simulink model "KalmanPrep"  (R2023b)
settings: Solver=FixedStepAuto  StartTime=0.0  StopTime=50  FixedStep=0.001  RelTol=1e-3
values from neighbouring files (symbols this model uses):
  A = [1, 0, Ts, 0 ... (first row only)    [Kal5Prep.m]    (also in KalPrep_mat.m = [1, Ts)
  B = [Ts, 0 ... (first row only)    [Kal5Prep.m]    (also in KalPrep_mat.m = [Ts; 0])
  bias = 0.5    [KalPrep_mat.m]
  C = [1, 0]    [KalPrep_mat.m]
  cov_ic = P0 * (1 + 2*rand)    [Kal5Prep.m]    (also in KalPrep_mat.m = eye(2) * alpha)
  eta1 = 0.002    [Kal5Prep.m]    (also in KalPrep_mat.m = deg2rad(1))
  eta2 = 0    [KalPrep_mat.m]
  eta_max = 0.4    [KalPrep_mat.m]
  G = eye(4) * Ts    [Kal5Prep.m]    (also in KalPrep_mat.m = [Ts 0)
  init_cond = [0; 0; 0.02; 0.01]    [Kal5Prep.m]    (also in KalPrep_mat.m = [pi/2; 5])
  K1 = 0.48    [KalPrep_mat.m]
  K2 = 0.16    [KalPrep_mat.m]
  pb = [0.5; 0.5]    [Kal5Prep.m]
  Q = eye(4)    [Kal5Prep.m]    (also in KalPrep_mat.m = [(sig1^2), 0)
  R = (eta1)^2    (= 4e-06)    [Kal5Prep.m]    (also in KalPrep_mat.m = (eta1)^2)
  sig1 = 0.005    [Kal5Prep.m]    (also in KalPrep_mat.m = 0.1)
  sig2 = 0.001    [Kal5Prep.m]    (also in KalPrep_mat.m = 0.2)
  Ts = 0.001    [Kal5Prep.m]    (also in KalPrep_mat.m)
  v0 = [1; 0]    [Kal5Prep.m]
libraries: dspsrcs4 x3
settings Model: Creator=fabio  LastModifiedBy=fabio

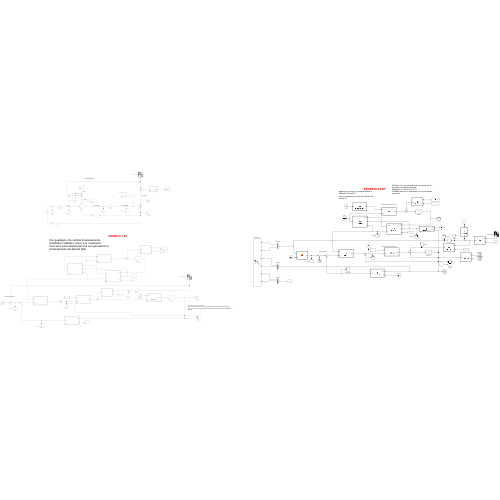
[thumbnail: Simulink's stored preview of the top-level diagram]
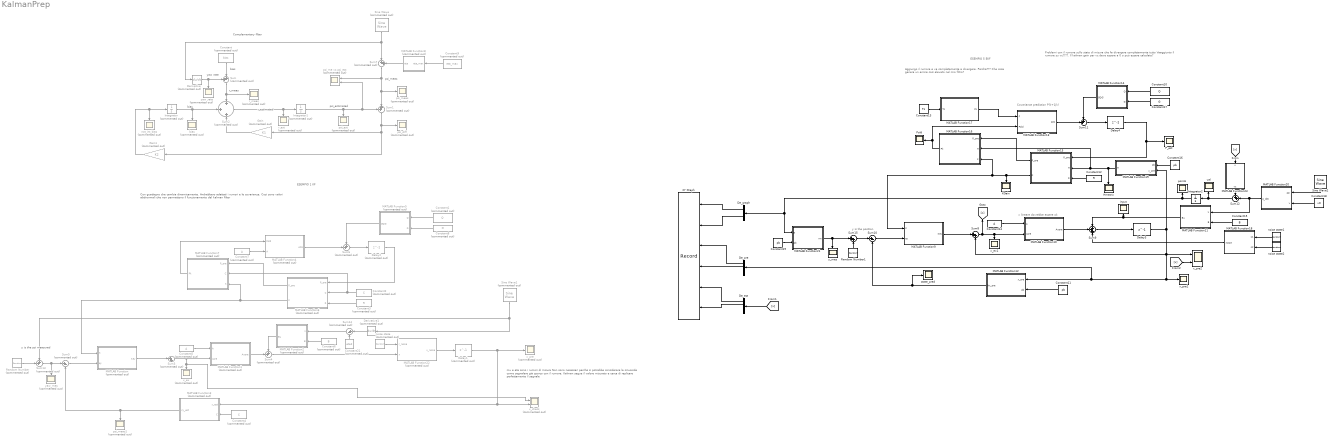
== system KalmanPrep ==
  note: Problemi con il rumore sullo stato di misura che fa divergere completamente tutto
      | Vaaggiunto il rumore su vc????.
      | Il kalman gain per vc deve essere a 0 o può essere calcolato?
  note: Aggiungo il rumore e va completamente a divergere. Perchè???
      | Che cosa genera un errore così elevato nel mio filtro?
  note: Complementary filter
  note: mu e eta sono i rumori di misura
      | Non sono necessari perchè si potrebbe considerare la sinusoide come segnalere già sporco con il rumore. Kalman segue il valore misurato e cerca di replicare perfettamente il segnale
  note: x lineare dovrebbe essere ok
  note: Covariance prediction P(k+1|k)
  note: ESEMPIO 5 EKF
  note: ESEMPIO 1 KF
  note: Con guadagno che cambia dinamicamente.
      | Andrebbero adattati i rumori e le covarianze.
      | Così sono valori abdnormali che non permettono il funzionamento del kalman filter
  note: y is the psi measured
  note: psi_meas
  note: yaw rate
  note: bias
  note: r_meas
  note: bias
  note: r_estimated
  note: psi_estimated
  note: y is the position
  Constant : Constant  Commented=on  Value=bias
  Constant1 : Constant  Commented=on  Value=Q
  Constant10 : Constant  Value=Q  VectorParams1D=off
  Constant11 : Constant  Value=pb  VectorParams1D=off
  Constant12 : Constant  Value=R
  Constant13 : Constant  Value=Ts
  Constant14 : Constant  Value=A  VectorParams1D=off
  Constant15 : Constant  Value=B  VectorParams1D=off
  Constant16 : Constant  Value=pb  VectorParams1D=off
  Constant17 : Constant  Value=G  VectorParams1D=off
  Constant18 : Constant  Value=v0  VectorParams1D=off
  Constant19 : Constant  Value=pb  VectorParams1D=off
  Constant2 : Constant  Commented=on  Value=C  VectorParams1D=off
  Constant21 : Constant  Commented=on  Value=eta2  VectorParams1D=off
  Constant3 : Constant  Commented=on  Value=R
  Constant4 : Constant  Commented=on  Value=C  VectorParams1D=off
  Constant5 : Constant  Commented=on  Value=A
  Constant6 : Constant  Commented=on  Value=B
  Constant7 : Constant  Commented=on  Value=A
  Constant8 : Constant  Commented=on  Value=G
  Constant9 : Constant  Commented=on  Value=eta_max
  De_est : Demux
  De_graph : Demux  Outputs=2
  De_pre : Demux
  Delay1 : Delay  Commented=on  DelayLength=1  InitialCondition=init_cond  UseCircularBuffer=on
  Delay2 : Delay  Commented=on  DelayLength=1  InitialCondition=cov_ic  UseCircularBuffer=on
  Delay3 : Delay  DelayLength=1  InitialCondition=init_cond  UseCircularBuffer=on
  Delay4 : Delay  DelayLength=1  InitialCondition=cov_ic  UseCircularBuffer=on
  Derivative : Derivative  Commented=on
  Derivative1 : Derivative  Commented=on
  Gain : Gain  Commented=on  Gain=K1
  Gain1 : Gain  Commented=on  Gain=K2
  Hmatrix : Scope
  Integrator : Integrator  Commented=on
  Integrator1 : Integrator  Commented=on
  Integrator2 : Integrator
  KGain : Scope
  MATLAB Function : MATLAB Function  Commented=on  TreatAsAtomicUnit=on
  MATLAB Function1 : MATLAB Function  Commented=on  TreatAsAtomicUnit=on
  MATLAB Function10 : MATLAB Function  TreatAsAtomicUnit=on
  MATLAB Function11 : MATLAB Function  TreatAsAtomicUnit=on
  MATLAB Function12 : MATLAB Function  TreatAsAtomicUnit=on
  MATLAB Function13 : MATLAB Function  TreatAsAtomicUnit=on
  MATLAB Function14 : MATLAB Function  TreatAsAtomicUnit=on
  MATLAB Function15 : MATLAB Function  TreatAsAtomicUnit=on
  MATLAB Function16 : MATLAB Function  TreatAsAtomicUnit=on
  MATLAB Function17 : MATLAB Function  TreatAsAtomicUnit=on
  MATLAB Function18 : MATLAB Function  TreatAsAtomicUnit=on
  MATLAB Function19 : MATLAB Function  TreatAsAtomicUnit=on
  MATLAB Function2 : MATLAB Function  Commented=on  TreatAsAtomicUnit=on
  MATLAB Function20 : MATLAB Function  TreatAsAtomicUnit=on
  MATLAB Function21 : MATLAB Function  TreatAsAtomicUnit=on
  MATLAB Function22 : MATLAB Function  Commented=on  TreatAsAtomicUnit=on
  MATLAB Function23 : MATLAB Function  TreatAsAtomicUnit=on
  MATLAB Function3 : MATLAB Function  Commented=on  TreatAsAtomicUnit=on
  MATLAB Function4 : MATLAB Function  Commented=on  TreatAsAtomicUnit=on
  MATLAB Function5 : MATLAB Function  Commented=on  TreatAsAtomicUnit=on
  MATLAB Function6 : MATLAB Function  Commented=on  TreatAsAtomicUnit=on
  MATLAB Function7 : MATLAB Function  Commented=on  TreatAsAtomicUnit=on
  MATLAB Function8 : MATLAB Function  Commented=on  TreatAsAtomicUnit=on
  MATLAB Function9 : MATLAB Function  TreatAsAtomicUnit=on
  P_est : Scope
  Pold : Scope
  Random Number : RandomNumber  Commented=on  Variance=eta1  SampleTime=Ts  VectorParams1D=off
  Random Number1 : RandomNumber  Variance=eta1  SampleTime=Ts
  Sine Wave : dspsrcs4/Sine Wave  Commented=on  Amplitude=1  Frequency=100  Phase=0  SampleMode=Discrete  OutComplex=Real  CompMethod=Trigonometric fcn  TableSize=Speed  SampleTime=1/1000  SamplesPerFrame=1  ResetState=Restart at time zero  OutputFrames=off  dataType=double  wordLen=16  udDataType=sfix(16)  fracBitsMode=Best precision  numFracBits=15  OutDataTypeStr=double  LastOutDataTypeStr=double
  Sine Wave1 : dspsrcs4/Sine Wave  Commented=on  Amplitude=1  Frequency=10  Phase=0  SampleMode=Discrete  OutComplex=Real  CompMethod=Trigonometric fcn  TableSize=Speed  SampleTime=1/1000  SamplesPerFrame=1  ResetState=Restart at time zero  OutputFrames=off  dataType=double  wordLen=16  udDataType=sfix(16)  fracBitsMode=Best precision  numFracBits=15  OutDataTypeStr=double  LastOutDataTypeStr=double
  Sine Wave2 : dspsrcs4/Sine Wave  Amplitude=1  Frequency=0.1  Phase=0  SampleMode=Discrete  OutComplex=Real  CompMethod=Trigonometric fcn  TableSize=Speed  SampleTime=1/1000  SamplesPerFrame=1  ResetState=Restart at time zero  OutputFrames=off  dataType=double  wordLen=16  udDataType=sfix(16)  fracBitsMode=Best precision  numFracBits=15  OutDataTypeStr=double  LastOutDataTypeStr=double
  Sum{,1,4,6,13} (5 alike) : Sum  Commented=on  Inputs=++|
  Sum10 : Sum  Inputs=|+-
  Sum11 : Sum  Inputs=++|
  Sum12 : Sum  Inputs=++|
  Sum14 : Sum  Commented=on  Inputs=|+-
  Sum15 : Sum  Inputs=|++
  Sum2 : Sum  Commented=on  Inputs=+||+||+
  Sum3 : Sum  Commented=on  Inputs=|++
  Sum5 : Sum  Commented=on  Inputs=|+-
  Sum7 : Sum  Commented=on  Inputs=|++
  Sum8 : Sum  Inputs=|++
  Sum9 : Sum  Inputs=+++
  XY Graph : Record  FileSettingsInternal="{\"entries\":[{\"content\":{\"excelSettings\":{\"content\":{},\"type\":\"Streamout.ExcelSettings\"}},\"type\":\"Streamout.FileSettingStorage\",\"uuid\":\"\"}],\"packageUris\":[\"http:\\/\\/schema.mathworks.com\\/mf0\\/streamout_blocks\\/R2020a\"],\"version\":\"1.0\"}"  Layout=[1 1]  SignalsInternal="{\"entries\":[{\"content\":{\"signals\":[{\"content\":{\"blockPath\":[],\"dimensions\":[1],\"domain\":\"\",\"lineColor\":\"#fe330a\",\"plots\":[ 1 ],\"port\":1,\"sid\":[\"\"],\"signalID\":1,\"signalName\":\"De_graph:1\"},\"type\":\"RecordBlkView.Signal\",\"uuid\":\"\"},{\"content\":{\"blockPath\":[],\"dimensions\":[1],\"domain\":\"\",\"lineColor\":\"#d95319\",\"plots\":[ 1 ],\"port\":2,\"sid\":[\"\"],\"signalID\":2,\"signalName\":\"De_graph:2\"},\"type\":\"RecordBlkView.Signal\",\"uuid\":\"\"},{\"content\":{\"blockPath\":[],\"dimensions\":[1],\"domain\":\"\",\"lineColor\":\"#22b573\",\"plots\":[ 1 ],\"port\":3,\"sid\":[\"\"],\"signalID\":3,\"signalName\":\"De_pre:1\"},\"type\":\"RecordBlkView.Signal\",\"uuid\":\"\"},{\"content\":{\"blockPath\":[],\"dimensions\":[1],\"domain\":\"\",\"lineColor\":\"#22b573\",\"plots\":[ 1 ],\"port\":4,\"sid\":[\"\"],\"signalID\":4,\"signalName\":\"De_pre:2\"},\"type\":\"RecordBlkView.Signal\",\"uuid\":\"\"},{\"content\":{\"blockPath\":[],\"dimensions\":[1],\"domain\":\"\",\"lineColor\":\"#4dbeee\",\"lineWidth\":2,\"plots\":[ 1 ],\"port\":5,\"sid\":[\"\"],\"signalID\":5,\"signalName\":\"De_est:1\"},\"type\":\"RecordBlkView.Signal\",\"uuid\":\"\"},{\"content\":{\"blockPath\":[],\"dimensions\":[1],\"domain\":\"\",\"lineColor\":\"#4dbeee\",\"plots\":[ 1 ],\"port\":6,\"sid\":[\"\"],\"signalID\":6,\"signalName\":\"De_est:2\"},\"type\":\"RecordBlkView.Signal\",\"uuid\":\"\"}]},\"type\":\"RecordBlkView.InputSignals\",\"uuid\":\"\"}],\"packageUris\":[\"http:\\/\\/schema.mathworks.com\\/mf0\\/streamout_blocks\\/R2020a\"],\"version\":\"1.0\"}"  VisualizationBindings="{\"xyplotplugin\":{\"info\":[{\"series\":[{\"bindingParametersList\":[{\"parameter\":\"X-Axis\",\"signalID\":3,\"signalName\":\"De_pre:1\"},{\"parameter\":\"Y-Axis\",\"signalID\":4,\"signalName\":\"De_pre:2\"}],\"seriesID\":0},{\"bindingParametersList\":[{\"parameter\":\"X-Axis\",\"signalID\":5,\"signalName\":\"De_est:1\"},{\"parameter\":\"Y-Axis\",\"signalID\":6,\"signalName\":\"De_est:2\"}],\"seriesID\":1},{\"bindingParametersList\":[{\"parameter\":\"X-Axis\",\"signalID\":1,\"signalName\":\"De_graph:1\"},{\"parameter\":\"Y-Axis\",\"signalID\":2,\"signalName\":\"De_graph:2\"}],\"seriesID\":2}],\"subplotID\":1}]}}"  CompatibilityTag=XY
  bias : Scope  Commented=on
  input : Scope
  noise state : RandomNumber  Commented=on  Variance=sig1  SampleTime=Ts
  noise state1 : RandomNumber  Variance=sig1  SampleTime=Ts
  noise state2 : RandomNumber  Variance=sig2  SampleTime=Ts
  not_int_bias : Scope  Commented=on
  points : Scope
  psi_diff : Scope  Commented=on
  psi_est : Scope  Commented=on
  psi_me vs psi_est : Scope  Commented=on  NumInputPorts=2
  psi_meas : Scope  Commented=on
  psi_meas1 : Scope  Commented=on
  r_est : Scope  Commented=on
  r_meas : Scope  Commented=on
  state_pred : Scope
  vel : Scope
  x_check : Scope  Commented=on  NumInputPorts=2
  x_ex : Scope  Commented=on
  x_ex1 : Scope
  x_pre : Scope  Commented=on
  x_pre1 : Scope
  x_pre2 : Scope  NumInputPorts=2
  y_mes : Scope
  yaw_mes : Scope  Commented=on
  yaw_rate : Scope  Commented=on
  wires:
  Derivative/1 -> yaw_rate/1, Sum/1
  Constant/1 -> Sum/2
  Sine Wave/1 -> Sum7/1, Derivative/1
  Sum/1 -> Sum2/1, r_meas/1
  Integrator/1 -> Sum2/2, bias/1
  Sum2/1 -> r_est/1, Integrator1/1
  Integrator1/1 -> psi_est/1, psi_me vs psi_est/2, Sum1/1
  Gain/1 -> Sum2/3
  Sum1/1 -> psi_diff/1, Gain1/1, Gain/1
  Gain1/1 -> not_int_bias/1, Integrator/1
  MATLAB Function/1(Key) -> Sum3/1
  Sum3/1 -> MATLAB Function1/2(xpre), x_check/1, x_ex/1
  MATLAB Function1/1(Axpre) -> Sum4/2
  MATLAB Function2/1(Bu) -> Sum4/1
  Sum5/1 -> MATLAB Function/2(ey)
  MATLAB Function3/1(cy_est) -> Sum5/2, psi_meas1/1
  MATLAB Function5/1(GQG) -> Sum6/1
  MATLAB Function4/1(APA) -> Sum6/2
  Delay2/1 -> MATLAB Function6/1("P_pre ")
  Sum6/1 -> Delay2/1
  Constant1/1 -> MATLAB Function5/1(Q)
  MATLAB Function6/2(K) -> MATLAB Function7/3(K), MATLAB Function/1(K)
  Constant2/1 -> MATLAB Function7/2(C), MATLAB Function6/2(C)
  Constant3/1 -> MATLAB Function6/3(R)
  MATLAB Function7/1(Pk) -> MATLAB Function4/1(Pold)
  Constant4/1 -> MATLAB Function3/2(C)
  Sine Wave1/1 -> Sum13/1, Derivative1/1
  Constant5/1 -> MATLAB Function1/1(A)
  Constant6/1 -> MATLAB Function2/2(B)
  Constant7/1 -> MATLAB Function4/2(A)
  Constant8/1 -> MATLAB Function5/2(G)
  MATLAB Function6/1(P_pre) -> MATLAB Function7/1(P_pre)
  Derivative1/1 -> Sum14/1
  Sum7/1 -> psi_me vs psi_est/1, Sum1/2, psi_meas/1
  Constant9/1 -> MATLAB Function8/1(eta_max)
  MATLAB Function8/1(eta) -> Sum7/2
  MATLAB Function17/1(Fk) -> MATLAB Function13/1(F)
  Delay3/1 -> x_pre1/1, De_pre/1, MATLAB Function12/1(x_pre), Sum8/2, x_pre2/1, MATLAB Function19/2(x_pre)
  Delay4/1 -> P_est/1, MATLAB Function15/1("P_pre ")
  MATLAB Function12/1(hx_pre) -> Sum10/2, state_pred/1
  Sum10/1 -> MATLAB Function9/2(ey)
  MATLAB Function19/1(H) -> MATLAB Function16/2(H), MATLAB Function15/2(H), Hmatrix/1
  Constant15/1 -> MATLAB Function11/2(B)
  Constant17/1 -> MATLAB Function14/2(G)
  MATLAB Function14/1(GQG) -> Sum11/1
  MATLAB Function13/1(FPF) -> Sum11/2
  Constant10/1 -> MATLAB Function14/1(Q)
  MATLAB Function10/1(Axpre) -> Sum9/2
  MATLAB Function16/1(Pk) -> Pold/1, MATLAB Function13/2(Pold)
  Constant14/1 -> MATLAB Function10/1(A)
  Sum9/1 -> Delay3/1
  MATLAB Function11/1(Bu) -> Sum9/1, input/1
  Constant12/1 -> MATLAB Function15/3(R)
  MATLAB Function15/2(K) -> KGain/1, MATLAB Function16/3(K), MATLAB Function9/1(K)
  Sum11/1 -> Delay4/1
  Sum8/1 -> MATLAB Function10/2(xpre), x_ex1/1, [x]
  MATLAB Function15/1(P_pre) -> MATLAB Function16/1(P_pre)
  MATLAB Function9/1(Key) -> Sum8/1
  Constant11/1 -> MATLAB Function12/2(pb)
  Constant13/1 -> MATLAB Function17/1(Ts)
  Constant16/1 -> MATLAB Function19/1(pb)
  Sine Wave2/1 -> MATLAB Function20/1(psi)
  MATLAB Function20/1(p_dot) -> MATLAB Function11/1(u), Sum12/2
  Integrator2/1 -> De_graph/1, MATLAB Function21/1(p), points/1
  Constant18/1 -> MATLAB Function20/2(v)
  MATLAB Function21/1(rm) -> Sum15/1, y_mes/1
  Constant19/1 -> MATLAB Function21/2(pb)
  Sum12/1 -> Integrator2/1, vel/1
  De_graph/2 -> XY Graph/2
  De_graph/1 -> XY Graph/1
  De_pre/1 -> XY Graph/3
  De_pre/2 -> XY Graph/4
  De_est/1 -> XY Graph/5
  De_est/2 -> XY Graph/6
  Sum13/1 -> yaw_mes/1, Sum5/1
  Random Number/1 -> Sum13/2
  Sum14/1 -> MATLAB Function2/1(u)
  Constant21/1 -> Sum14/2
  Sum4/1 -> MATLAB Function22/2(x)
  MATLAB Function22/1(x_noise) -> Delay1/1
  noise state/1 -> MATLAB Function22/1(r_noise)
  Delay1/1 -> MATLAB Function3/1(y_est), x_check/2, x_pre/1
  Sum15/1 -> Sum10/1
  Random Number1/1 -> Sum15/2
  MATLAB Function18/1(noise) -> Sum9/3
  noise state1/1 -> MATLAB Function18/1(s1)
  noise state2/1 -> MATLAB Function18/2(s2)
  MATLAB Function23/1(vc) -> Sum12/1
  [x] -> MATLAB Function23/1(x)
  [x] -> De_est/1
  [x] -> x_pre2/2

== matlab function KalmanPrep/MATLAB Function1 ==
  data: A input; xpre input; Axpre output
function Axpre= Amatrix(A, xpre)
    Axpre = A * xpre;

== matlab function KalmanPrep/MATLAB Function12 ==
  data: x_pre input; hx_pre output; pb input
function hx_pre = OutputPre(x_pre, pb)
    hx_pre = norm((x_pre(1:2) - pb));

== matlab function KalmanPrep/MATLAB Function13 ==
  data: F input; Pold input; FPF output
function FPF = Fmatrix(F, Pold)
    FPF = F*Pold*(F');

== matlab function KalmanPrep/MATLAB Function14 ==
  data: Q input; GQG output; G input
function GQG = GmatrixQ(Q, G)
    GQG = G*Q*(G');

== matlab function KalmanPrep/MATLAB Function15 ==
  data: P_pre output; P_pre input; H input; K output; R input
function [P_pre, K] = KalmanGain(P_pre, H, R)
    K = (P_pre*(H'))*pinv((H*P_pre*(H') + R)); 
    % Bayas do not have to update??
    % K(3) = 0  ; K(4) = 0;

== matlab function KalmanPrep/MATLAB Function16 ==
  data: P_pre input; H input; Pk output; K input
function Pk = PkComp(P_pre, H, K)
    s = size((K*H), 1); % Controlla che funzioni
    I = eye(s); 
    Pk = (I - K*H)*P_pre;

== matlab function KalmanPrep/MATLAB Function9 ==
  data: K input; ey input; Key output
function Key = GainMult(K, ey)
    Key = K*ey;

== matlab function KalmanPrep/MATLAB Function17 ==
  data: Fk output; Ts input
function Fk = DynamicJacobian(Ts)
    Fk = eye(4);
    Fk(1:2, 3:4) = Ts * eye(2);

== matlab function KalmanPrep/MATLAB Function18 ==
  data: s1 input; noise output; s2 input
function noise = StateNoise(s1, s2) 
    noise = [s1, s1, s2, s2]';

== matlab function KalmanPrep/MATLAB Function19 ==
  data: pb input; x_pre input; H output
function H = HComputation(pb, x_pre)
    Ht = ((x_pre(1:2) - pb))' / (norm(x_pre(1:2) - pb));
    H = [Ht 0 0];

== matlab function KalmanPrep/MATLAB Function20 ==
  data: psi input; p_dot output; v input
function p_dot = InputComp(psi, v) 
    R = [cos(psi) -sin(psi);
         sin(psi) cos(psi)];
    p_dot = R * v;

== matlab function KalmanPrep/MATLAB Function ==
  data: K input; ey input; Key output
function Key = GainMult(K, ey)
    Key = K*ey; % 2x1

== matlab function KalmanPrep/MATLAB Function21 ==
  data: p input; pb input; rm output
function rm = Ymeasured(p, pb) 
    rm = norm(p - pb);

== matlab function KalmanPrep/MATLAB Function22 ==
  data: r_noise input; x input; x_noise output
function x_noise = StateNoise (r_noise, x)
    x_noise = zeros(2,1);
    x_noise(1) = x(1) + r_noise;

== matlab function KalmanPrep/MATLAB Function23 ==
  data: x input; vc output
function vc = VcExtraction(x) 
    vc = x(3:4);

== matlab function KalmanPrep/MATLAB Function2 ==
  data: u input; Bu output; B input
function Bu = Bmatrix(u, B) 
    Bu = B * u;

== matlab function KalmanPrep/MATLAB Function3 ==
  data: y_est input; cy_est output; C input
function cy_est = Cmatrix(y_est, C)
    cy_est = C * y_est; % 1x1

== matlab function KalmanPrep/MATLAB Function4 ==
  data: Pold input; APA output; A input
function APA = Amatrix(Pold, A)
    APA = A*Pold*(A');

== matlab function KalmanPrep/MATLAB Function5 ==
  data: Q input; GQG output; G input
function GQG = GmatrixQ(Q, G)
    GQG = G*Q*(G');

== matlab function KalmanPrep/MATLAB Function6 ==
  data: P_pre output; P_pre input; C input; K output; R input
function [P_pre, K] = KalmanGain(P_pre, C, R)
    K = zeros(2,1);
    K = (P_pre*(C'))*pinv((C*P_pre*(C') + R)); % 2x1
    K(2) = 0;

== matlab function KalmanPrep/MATLAB Function7 ==
  data: P_pre input; C input; Pk output; K input
function Pk = PkComp(P_pre, C, K)
    I = eye(2); % mod con dimesnione K*C
    Pk = (I - K*C)*P_pre; % 2x2 ok

== matlab function KalmanPrep/MATLAB Function8 ==
  data: eta_max input; eta output
function eta = fcn(eta_max)
    eta = 0.5 * rand;

== matlab function KalmanPrep/MATLAB Function10 ==
  data: A input; xpre input; Axpre output
function Axpre= Amatrix(A, xpre)
    Axpre = A * xpre;

== matlab function KalmanPrep/MATLAB Function11 ==
  data: u input; Bu output; B input
function Bu = Bmatrix(u, B) 
    Bu = B * u;
